simulink subsystem "Kinematika_B"  (R2024b)
settings: Solver=VariableStepAuto  StartTime=0.0  StopTime=10.0  RelTol=1e-3
values from neighbouring files (symbols this model uses):
  c = 0    [D1script.m]    (also in disp.mat; onlabscript.m)
settings Model: Creator=Asus  LastModifiedBy=Asus

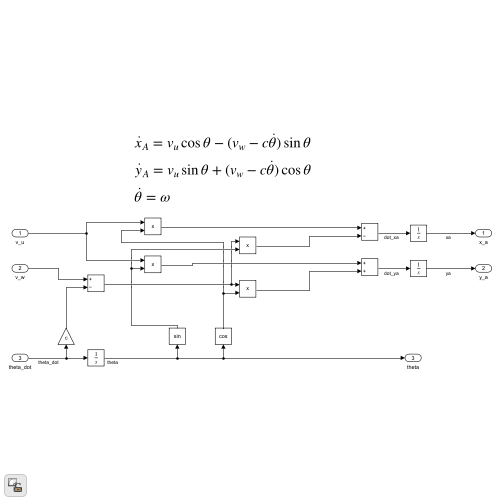
[thumbnail: Simulink's stored preview of the top-level diagram]
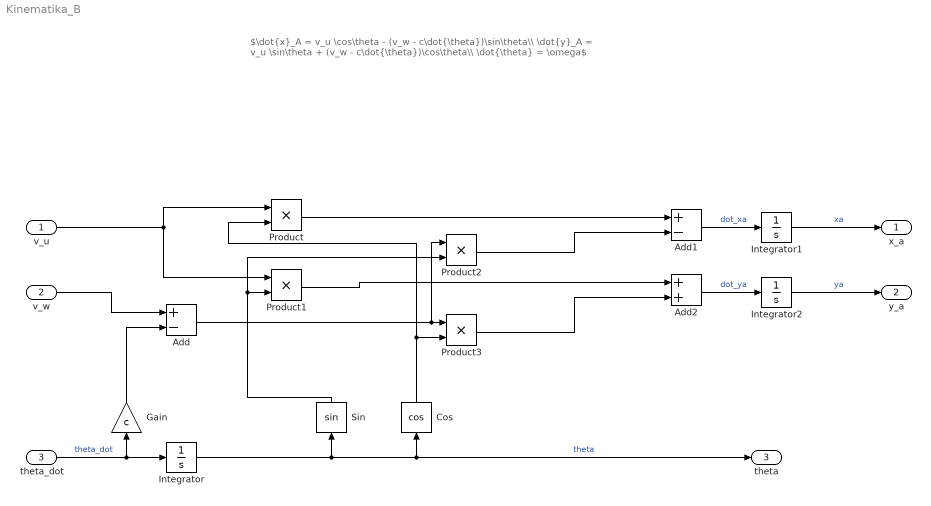
== system Kinematika_B ==
  note: $\dot{x}_A = v_u \cos\theta - (v_w - c\dot{\theta})\sin\theta\\ \dot{y}_A = v_u \sin\theta + (v_w - c\dot{\theta})\cos\theta\\ \dot{\theta} = \omega$
  v_u : Inport
  v_w : Inport  Port=2
  theta_dot : Inport  Port=3
  Add : Sum  Inputs=+-
  Add1 : Sum  Inputs=+-
  Add2 : Sum
  Cos : Trigonometry  Operator=cos
  Gain : Gain  Gain=c
  Integrator : Integrator
  Integrator1 : Integrator
  Integrator2 : Integrator
  Product{,1..3} (4 alike) : Product
  Sin : Trigonometry
  x_a : Outport
  y_a : Outport  Port=2
  theta : Outport  Port=3
  wires:
  theta_dot/1 -> Integrator/1, Gain/1  "theta_dot"
  Integrator/1 -> theta/1, Cos/1, Sin/1  "theta"
  Gain/1 -> Add/2
  v_w/1 -> Add/1
  v_u/1 -> Product/1, Product1/1
  Sin/1 -> Product1/2, Product2/2
  Cos/1 -> Product/2, Product3/2
  Product/1 -> Add1/1
  Add/1 -> Product3/1, Product2/1
  Product1/1 -> Add2/1
  Add1/1 -> Integrator1/1  "dot_xa"
  Integrator1/1 -> x_a/1  "xa"
  Add2/1 -> Integrator2/1  "dot_ya"
  Integrator2/1 -> y_a/1  "ya"
  Product2/1 -> Add1/2
  Product3/1 -> Add2/2
